simulink model "ANC_model"  (R2026a)
settings: Solver=FixedStepDiscrete  StopTime=5  FixedStep=1/8000
libraries: dspadpt3 x1
settings Model: Creator=ojasv  LastModifiedBy=ojasv

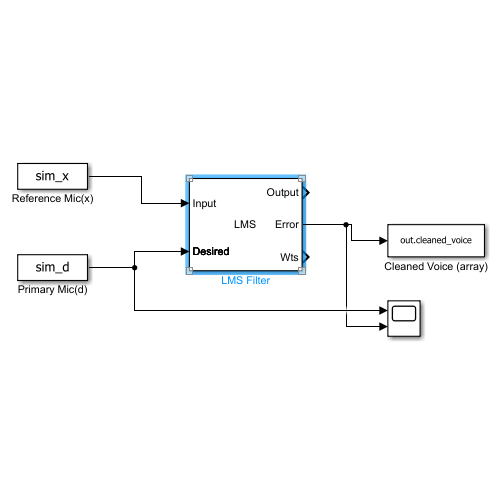
[thumbnail: Simulink's stored preview of the top-level diagram]
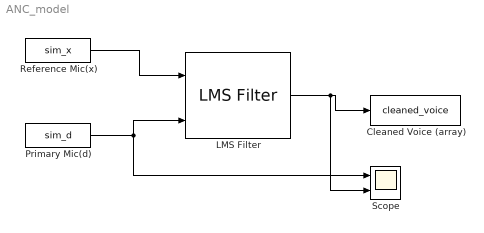
== system ANC_model ==
  Cleaned Voice (array) : ToWorkspace  VariableName=cleaned_voice  SampleTime=-1
  LMS Filter : dspadpt3/LMS Filter  Algo=LMS  L=64  stepflag=Dialog  mu=0.001  leakage=1.0  ic=0  Adapt=off  resetflag=None  weights=on  addnparflag=off  roundingMode=Floor  overflowMode=off
  Primary Mic(d) : FromWorkspace  VariableName=sim_d  SampleTime=1/8000
  Reference Mic(x) : FromWorkspace  VariableName=sim_x  SampleTime=1/8000
  Scope : Scope  NumInputPorts=2
      settings: ActiveDisplayYMinimum=-16.599655772595643  ActiveDisplayYMaximum=19.292935661267403
  wires:
  Reference Mic(x)/1 -> LMS Filter/1
  Primary Mic(d)/1 -> Scope/1, LMS Filter/2
  LMS Filter/2 -> Cleaned Voice (array)/1, Scope/2
